simulink model "system"  (Simulink 10.0)
settings: Solver=FixedStepDiscrete  StartTime=0.0  StopTime=tend  RelTol=1e-3  EnableMultiTasking=on
values from neighbouring files (symbols this model uses):
  c1o = 0.7    [zad1.m]    (also in zad2.m; zad3.m; zad4.m; zad5.m)
  f = 0.025    [zad1.m]    (also in zad2.m; zad3.m; zad4.m; zad5.m)
  Td = 1500    [zad1.m]    (also in zad2.m; zad3.m = 500; zad4.m; zad5.m = 500)
  Tp = 0.1    [zad1.m]    (also in zad2.m; zad3.m; zad4.m; zad5.m)
libraries: simulink x2
settings Model: Creator=szymo  LastModifiedBy=szymo
settings SolverCC: AutoInsertRateTranBlk=on
settings DataIOCC: LimitDataPoints=on  SignalLoggingSaveFormat=ModelDataLogs
settings OptimizationCC: InitFltsAndDblsToZero=on
settings DebuggingCC: SaveWithParameterizedLinksMsg=none  SignalResolutionControl=TryResolveAllWithWarning  SolverPrmCheckMsg=warning  MultiTaskDSMMsg=warning  MultiTaskCondExecSysMsg=none  FcnCallInpInsideContextMsg=warning
settings SFSimCC: SimUseLocalCustomCode=on  CustomCodeUndefinedFunction=FilterOut
settings RTWCC: RTWUseLocalCustomCode=on
settings GRTTargetCC: TargetFcnLib=ansi_tfl_tmw.mat

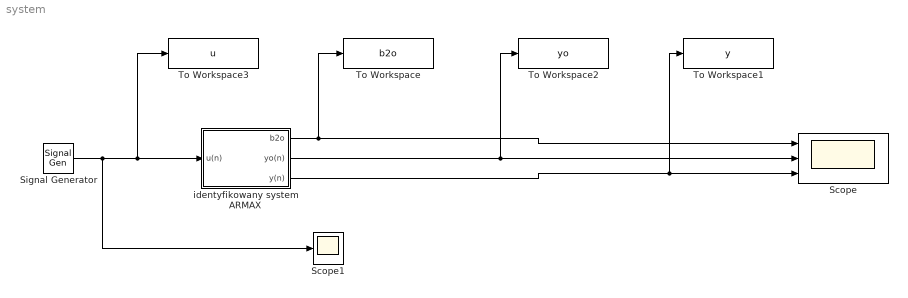
== system system ==
  Scope : Scope  NumInputPorts=3
  Scope1 : Scope
  Signal Generator : SignalGenerator  WaveForm=square  Frequency=f
  To Workspace : ToWorkspace  VariableName=b2o  SaveFormat=Timeseries  SampleTime=-1
  To Workspace1 : ToWorkspace  VariableName=y  SaveFormat=Timeseries  SampleTime=-1
  To Workspace2 : ToWorkspace  VariableName=yo  SaveFormat=Timeseries  SampleTime=-1
  To Workspace3 : ToWorkspace  VariableName=u  SaveFormat=Timeseries  SampleTime=-1
  identyfikowany system ARMAX : Subsystem
  wires:
  identyfikowany system ARMAX/2(yo(n)) -> To Workspace2/1, Scope/2
  identyfikowany system ARMAX/1(b2o) -> To Workspace/1, Scope/1
  identyfikowany system ARMAX/3(y(n)) -> To Workspace1/1, Scope/3
  Signal Generator/1 -> Scope1/1, To Workspace3/1, identyfikowany system ARMAX/1(u(n))

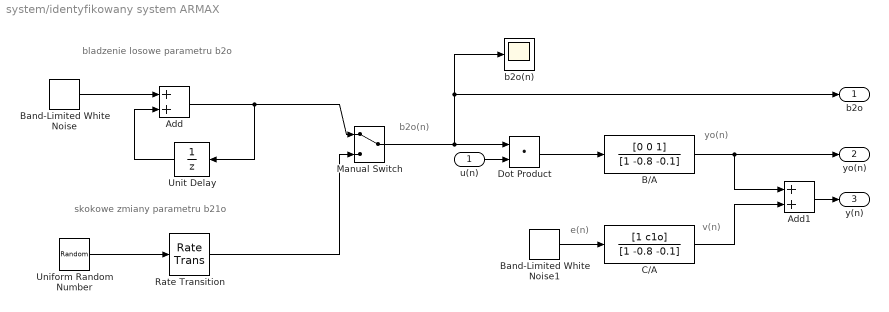
== system system/identyfikowany system ARMAX ==
  note: e(n)
  note: v(n)
  note: yo(n)
  note: b2o(n)
  note: skokowe zmiany parametru b21o
  note: bladzenie losowe parametru b2o
  u(n) : Inport
  Add : Sum
  Add1 : Sum
  B/A : DiscreteFilter  Numerator=[0 0 1]  Denominator=[1 -0.8 -0.1]  SampleTime=Tp
  Band-Limited White Noise : simulink/Sources/Band-Limited White Noise  Cov=[0.00001*Tp]  Ts=Tp  seed=[23341]
  Band-Limited White Noise1 : simulink/Sources/Band-Limited White Noise  Cov=[0.001*Tp]  Ts=Tp  seed=[23341]
  C/A : DiscreteFilter  Numerator=[1 c1o]  Denominator=[1 -0.8 -0.1]  SampleTime=Tp
  Dot Product : DotProduct  InputSameDT=on  OutDataTypeStr=Inherit: Inherit via internal rule
  Manual Switch : ManualSwitch
  Rate Transition : RateTransition  InitialCondition=0.5  OutPortSampleTime=Tp
  Uniform Random Number : UniformRandomNumber  Minimum=0.1  Maximum=0.8  Seed=2  SampleTime=Td
  Unit Delay : UnitDelay  SampleTime=Tp
  b2o(n) : Scope
  b2o : Outport
  yo(n) : Outport  Port=2
  y(n) : Outport  Port=3
  wires:
  Band-Limited White Noise/1 -> Add/1
  Add/1 -> Unit Delay/1, Manual Switch/1
  Unit Delay/1 -> Add/2
  Uniform Random Number/1 -> Rate Transition/1
  Rate Transition/1 -> Manual Switch/2
  Manual Switch/1 -> Dot Product/1, b2o/1, b2o(n)/1
  Dot Product/1 -> B/A/1
  C/A/1 -> Add1/2
  B/A/1 -> Add1/1, yo(n)/1
  Band-Limited White Noise1/1 -> C/A/1
  u(n)/1 -> Dot Product/2
  Add1/1 -> y(n)/1
